simulink model "untitled1"  (R2025b)
settings: Solver=FixedStepAuto  StartTime=0.0  StopTime=170000  FixedStep=1  RelTol=1e-3
values from neighbouring files (symbols this model uses):
  dx0 = [.05; .05; .05]    [dynamics_setup.m]
  Ib = [Ixx Ixy Izx ... (first row only)    [dynamics_setup.m]
  Ibinv = Ib^-1    [dynamics_setup.m]
  q0 = q0/norm(q0)    [dynamics_setup.m]
  R0 = quat2rotm([q0(4) q0(1) q0(2) q0(3)])    [dynamics_setup.m]
libraries: matrix_library x1
settings Model: Creator=Zargai  LastModifiedBy=Zargai
settings RTWCC: GenCodeOnly=on

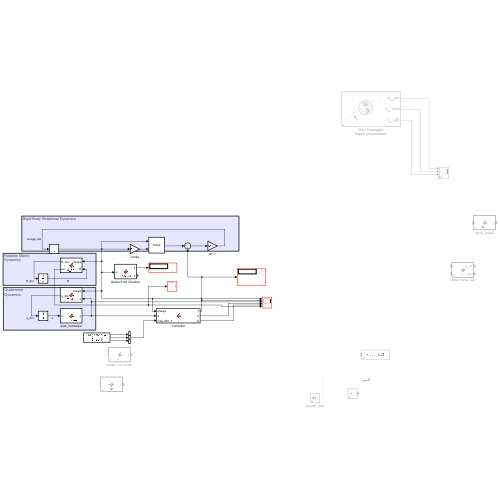
[thumbnail: Simulink's stored preview of the top-level diagram]
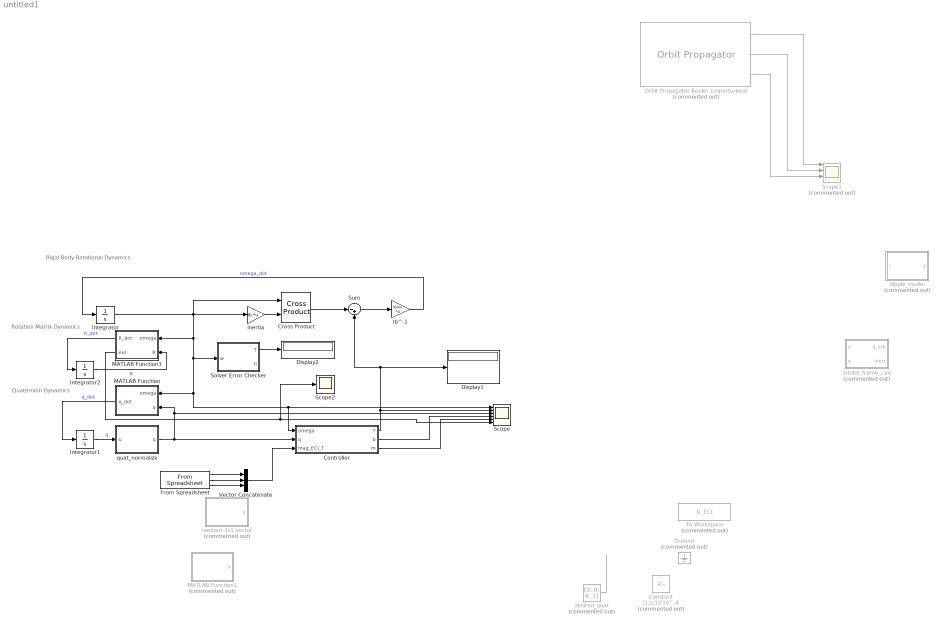
== system untitled1 ==
  note: Rotation Matrix
      | Dynamics
  note: Quaternion
      | Dynamics
  note: Rigid Body Rotational Dynamics
  Constant : Constant  Commented=on  Value=[1;1;1]*10^-4
  Controller : MATLAB Function  TreatAsAtomicUnit=on
  Cross Product : matrix_library/Cross Product
  Display1 : Display
  Display2 : Display
  From Spreadsheet : FromSpreadsheet  FileName=magdata.xlsx
  Ground : Ground  Commented=on
  Ib^-1 : Gain  Gain=Ibinv  Multiplication=Matrix(K*u)
  Integrator : Integrator  InitialCondition=dx0
  Integrator1 : Integrator  InitialCondition=q0
  Integrator2 : Integrator  InitialCondition=R0
  MATLAB Function : MATLAB Function  TreatAsAtomicUnit=on
  MATLAB Function1 : MATLAB Function  Commented=on  TreatAsAtomicUnit=on
  MATLAB Function3 : MATLAB Function  TreatAsAtomicUnit=on
  Orbit Propagator Kepler (unperturbed) : OrbitPropagator  Commented=on  semiMajorAxis=6968137  inclination=97.7496  raan=90  argPeriapsis=0  inertialPosition=[3649700.0 3308200.0 -4676600.0]  inertialVelocity=[-2750.8 6666.4 2573.4]  fixedPosition=[-4142689.0 -2676864.7 -4669861.6]  fixedVelocity=[1452.7 -6720.7 2568.1]  customR=3396200  customMu=4.305e13  customJ2=1.0826269e-03  customOmega=4.06125949e-3
  Scope : Scope  NumInputPorts=6
      settings: ActiveDisplayYMinimum=-4.340875855178699  ActiveDisplayYMaximum=4.9307851291899176
  Scope1 : Scope  Commented=on  NumInputPorts=4
      settings: ActiveDisplayYMinimum=-8.78056449714E+6  ActiveDisplayYMaximum=8.64689677459E+6
  Scope2 : Scope
      settings: ActiveDisplayYMinimum=-3.9269892667285857  ActiveDisplayYMaximum=3.9269862026038229  YLabel=Euler Angles (radians)  DataLoggingVariableName=ScopeData2
  Solver Error Checker : MATLAB Function  TreatAsAtomicUnit=on
  Sum : Sum  Inputs=|-+
  To Workspace : ToWorkspace  Commented=on  VariableName=b_ECI  SaveFormat=Timeseries  SampleTime=-1
  Vector Concatenate : Concatenate  NumInputs=3
  desired_quat : Constant  Commented=on  Value=[0; 0; 0; 1]
  dipole_model : MATLAB Function  Commented=on  TreatAsAtomicUnit=on
  inertia : Gain  Gain=Ib  Multiplication=Matrix(K*u)
  orbital_frame_calc : MATLAB Function  Commented=on  TreatAsAtomicUnit=on
  quat_normalize : MATLAB Function  TreatAsAtomicUnit=on
  random 3x1 vector : MATLAB Function  Commented=on  TreatAsAtomicUnit=on
  wires:
  Integrator/1 -> inertia/1, MATLAB Function3/1(omega), Solver Error Checker/1(w), Controller/1(omega), Scope/1, MATLAB Function/1(omega), Cross Product/1
  MATLAB Function/1(q_dot) -> Integrator1/1  "q_dot"
  Integrator1/1 -> quat_normalize/1(u)  "q"
  Ib^-1/1 -> Integrator/1  "omega_dot"
  inertia/1 -> Cross Product/2
  Cross Product/1 -> Sum/1
  Controller/1(T) -> Sum/2, Display1/1, Scope/2
  Sum/1 -> Ib^-1/1
  From Spreadsheet/1 -> Vector Concatenate/1
  From Spreadsheet/3 -> Vector Concatenate/3
  From Spreadsheet/2 -> Vector Concatenate/2
  desired_quat/1 -> ?
  Solver Error Checker/1(T) -> Display2/1
  Controller/2(b) -> Scope/4
  Controller/3(m) -> Scope/5
  Orbit Propagator Kepler (unperturbed)/1 -> Scope1/1
  Orbit Propagator Kepler (unperturbed)/2 -> Scope1/2
  Orbit Propagator Kepler (unperturbed)/3 -> Scope1/3
  quat_normalize/1(q) -> MATLAB Function/2(q), Scope/3, Controller/2(q)
  Integrator2/1 -> MATLAB Function3/2(R)  "R"
  MATLAB Function3/1(R_dot) -> Integrator2/1  "R_dot"
  MATLAB Function3/2(eul) -> Scope2/1, Scope/6
  Vector Concatenate/1 -> Controller/3(mag_ECI_T)

== matlab function untitled1/MATLAB Function1 ==
  data: y output
function y = fcn()

y = rand(3, 1) * 10^-4;

== matlab function untitled1/MATLAB Function ==
  data: omega input; q input; q_dot output
function q_dot = Q_dot(omega, q)

% Reference Crassidis Ch. 7.1

% skew = [0 -omega(3) omega(2);
%     omega(3) 0 -omega(1);
%     -omega(2) omega(1) 0];

% q_dot = .5* [-skew omega;
%     -omega' 0]* q;

q_dot = .5 * quat_cross_mult([omega; 0], q);

== matlab function untitled1/quat_normalize ==
  data: u input; q output
function q = q_norm(u)

q = u/norm(u);

== matlab function untitled1/Solver Error Checker ==
  data: w input; T output; h output
function [T, h] = checker(w)

Ixx = .03293;
Iyy = .13199;
Izz = .13943;
Ixy = .00005;
Iyz = -.00016;
Izx = -.00014;

Ib = [Ixx Ixy Izx;
    Ixy Iyy Iyz;
    Izx Iyz Izz];

T = w'*Ib*w;
h = norm(Ib*w);

== matlab function untitled1/dipole_model ==
  data: r input; y output
function y = fcn(r)
Bo = 3.12*10^-5;
r_earth = 6370000;
[az, el, r] = cart2sph(r(1), r(2), r(3));
colat = 90 - el;
br = -2*Bo*(r_earth/norm(r))^3*cos(colat); 
blat = -Bo*(r_earth/norm(r))^3*cos(colat); 

y = u;

== matlab function untitled1/random 3x1 vector ==
  data: y output
function y = fcn()

y = rand(3,1);

== matlab function untitled1/Controller ==
  data: omega input; T output; q input; mag_ECI_T input; b output; m output
function [T,b,m] = C(omega, q, mag_ECI_T)
Kd = .0001; % Pick a Kd
%Kp = .02*(50+Kd)^2; % Ballpark formula to attempt to obtain critical damping

Kp = .00001;

bq = quat_cross_mult(q, quat_cross_mult( [mag_ECI_T; 0] , quat_inv(q))); % Embed mag_ECI into quat and Transform from ECI to Body frame
b = bq(1:3); % Retrieve vector part

% debugging statement

omega_d = [0; 0; 0];
qd = [13; -123; 53; -43];
qd = qd/norm(qd);
omega_e = omega - omega_d;

qe = quat_cross_mult( q, quat_inv(qd) ); % Eqn 7.2 in Crassidis

Td = - Kp * sign(qe(4)) * qe(1:3) - Kd * omega_e(1:3); % Pd on error quaternion vector and rates. Included shortest angle rotation with sign(qe(4))

% Spin axis simulation

%Td = - Kp * qe(2:3) - Kd * omega_e(2:3); % Pd on error quaternion vector and rates. Included shortest angle rotation with sign(qe(4))
%Td = [0; Td];

m = cross(b, Td)/norm(b)^2;

% Saturate coils

m_max = [0.2; 0.2; 0.1];
m_max = [2000; 2000; 1000];

m = min(max(m, -m_max), m_max);

T = cross(m, b);

== matlab function untitled1/MATLAB Function3 ==
  data: omega input; R_dot output; R input; eul output
function [R_dot, eul] = R_dot(omega, R)

skew = [0 -omega(3) omega(2);
    omega(3) 0 -omega(1);
    -omega(2) omega(1) 0];

R_dot = R*skew;
eul = rotm2eul(R);

== matlab function untitled1/orbital_frame_calc ==
  data: x input; q_orb output; v input; inert output
function [q_orb,inert]= fcn(x, v)

nadir = -x/norm(x);
q_orb/inert =
